simulink model "Combine4_Model"  (R2023a)
settings: Solver=VariableStepAuto  StartTime=0.0  StopTime=10.0  RelTol=1e-3
libraries: NSA_DEVS_SINKS_ATOMIC x5, NSA_DEVS_SOURCES_ATOMIC x4, NSA_DEVS_ROUTING_ATOMIC x1, NSA_DEVS_LOGISTICS_ATOMIC x1
settings Model: Creator=david  LastModifiedBy=david

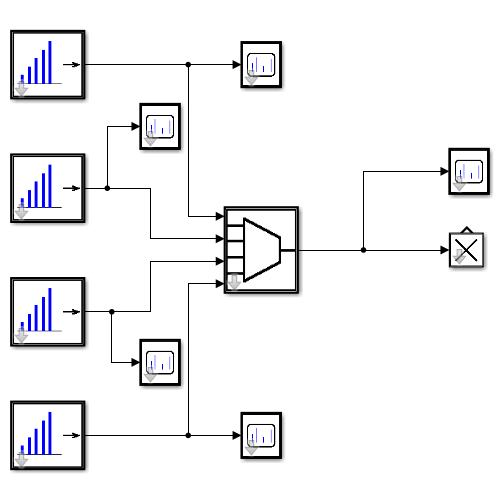
[thumbnail: Simulink's stored preview of the top-level diagram]
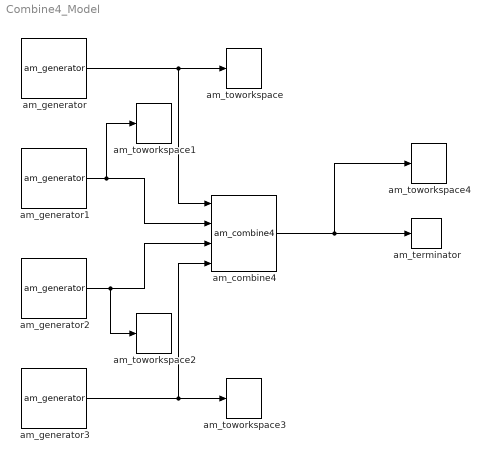
== system Combine4_Model ==
  am_combine4 : NSA_DEVS_ROUTING_ATOMIC/am_combine4  tD=[0,10]  tau=[0,10]  debug=0
      settings: SourceProductName=NSA_DEVS
  am_generator : NSA_DEVS_SOURCES_ATOMIC/am_generator  tG=1  n0=1  nG=100  tau=[0,1]  debug=0
      settings: SourceProductName=NSA_DEVS
  am_generator1 : NSA_DEVS_SOURCES_ATOMIC/am_generator  tG=2  n0=21  nG=100  tau=[0,1]  debug=0
      settings: SourceProductName=NSA_DEVS
  am_generator2 : NSA_DEVS_SOURCES_ATOMIC/am_generator  tG=3  n0=41  nG=100  tau=[0,1]  debug=0
      settings: SourceProductName=NSA_DEVS
  am_generator3 : NSA_DEVS_SOURCES_ATOMIC/am_generator  tG=3.5  n0=12  nG=100  tau=[0,1]  debug=0
      settings: SourceProductName=NSA_DEVS
  am_terminator : NSA_DEVS_LOGISTICS_ATOMIC/am_terminator  tau=[0,1]  debug=0
      settings: SourceProductName=NSA_DEVS
  am_toworkspace : NSA_DEVS_SINKS_ATOMIC/am_toworkspace  varname="\"gen1Out\""  t0=0  format="\"vector\""  tau=[0,1]  debug=0
      settings: SourceProductName=NSA_DEVS
  am_toworkspace1 : NSA_DEVS_SINKS_ATOMIC/am_toworkspace  varname="\"gen2Out\""  t0=0  format="\"vector\""  tau=[0,1]  debug=0
      settings: SourceProductName=NSA_DEVS
  am_toworkspace2 : NSA_DEVS_SINKS_ATOMIC/am_toworkspace  varname="\"gen3Out\""  t0=0  format="\"vector\""  tau=[0,1]  debug=0
      settings: SourceProductName=NSA_DEVS
  am_toworkspace3 : NSA_DEVS_SINKS_ATOMIC/am_toworkspace  varname="\"gen4Out\""  t0=0  format="\"vector\""  tau=[0,1]  debug=0
      settings: SourceProductName=NSA_DEVS
  am_toworkspace4 : NSA_DEVS_SINKS_ATOMIC/am_toworkspace  varname="\"combOut\""  t0=0  format="\"vector\""  tau=[0,1]  debug=0
      settings: SourceProductName=NSA_DEVS
  wires:
  am_generator1/1 -> am_toworkspace1/1, am_combine4/2
  am_generator2/1 -> am_toworkspace2/1, am_combine4/3
  am_generator/1 -> am_toworkspace/1, am_combine4/1
  am_generator3/1 -> am_toworkspace3/1, am_combine4/4
  am_combine4/1 -> am_toworkspace4/1, am_terminator/1
